simulink model "object"  (R2014a)
settings: Solver=ode45  StartTime=0.0  StopTime=T_sim  FixedStep=0.005  RelTol=1e-3
values from neighbouring files (symbols this model uses):
  Kp = 342.102792836    [all_data.mat]    (also in set_controller_MO.m = Ti/(2*num(end)*Tsig); set_controller_SO.m = T0/(2*K*Tsigma))
  T_sim = 10    [MO_test.m]    (also in SO_test.m; all_data.mat)
  Ti = 0.00201814300939    [all_data.mat]    (also in set_controller_MO.m = T2; set_controller_SO.m = 4*Tsigma)
libraries: cstblocks x1, simulink x1
settings Model: Creator=Gracex  LastModifiedBy=Gracex
settings DebuggingCC: SolverPrmCheckMsg=none

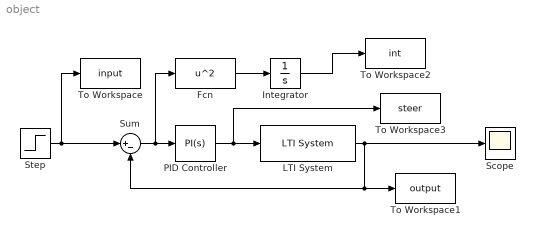
== system object ==
  Fcn : Fcn  Expr=u^2
  Integrator : Integrator
  LTI System : cstblocks/LTI System  sys=G_s  IC=[]
  PID Controller : simulink/Continuous/PID Controller  Controller=PI  TimeDomain=Continuous-time  SampleTime=1  IntegratorMethod=Forward Euler  FilterMethod=Forward Euler  Form=Ideal  P=Kp  I=1/Ti  D=0  N=100  InitialConditionSource=internal  InitialConditionForIntegrator=0  InitialConditionForFilter=0  ExternalReset=none  LimitOutput=off  UpperSaturationLimit=inf  LowerSaturationLimit=-inf  LinearizeAsGain=on  AntiWindupMode=none  Kb=1  TrackingMode=off  Kt=1  PParamMin=[]  PParamMax=[]  IParamMin=[]  IParamMax=[]  DParamMin=[]  DParamMax=[]  NParamMin=[]  NParamMax=[]  KbParamMin=[]  KbParamMax=[]  KtParamMin=[]  KtParamMax=[]  POutMin=[]  POutMax=[]  IOutMin=[]  IOutMax=[]  DOutMin=[]  DOutMax=[]  NOutMin=[]  NOutMax=[]  KbOutMin=[]  KbOutMax=[]  KtOutMin=[]  KtOutMax=[]  IntegratorOutMin=[]  IntegratorOutMax=[]  FilterOutMin=[]  FilterOutMax=[]  SumOutMin=[]  SumOutMax=[]  SumI1OutMin=[]  SumI1OutMax=[]  SumI2OutMin=[]  SumI2OutMax=[]  SumI3OutMin=[]  SumI3OutMax=[]  SumDOutMin=[]  SumDOutMax=[]  SaturationOutMin=[]  SaturationOutMax=[]  IntegratorContinuousStateAttributes=''  IntegratorStateMustResolveToSignalObject=off  IntegratorRTWStateStorageClass=Auto  FilterContinuousStateAttributes=''  FilterStateMustResolveToSignalObject=off  FilterRTWStateStorageClass=Auto
  Scope : Scope
  Step : Step  Time=T_sim/20  SampleTime=0
  Sum : Sum  Inputs=|+-
  To Workspace : ToWorkspace  VariableName=input  SaveFormat=Structure With Time  SampleTime=-1
      settings: Save2DSignal=2-D array (concatenate along first dimension)
  To Workspace1 : ToWorkspace  VariableName=output  SaveFormat=Structure With Time  SampleTime=-1
      settings: Save2DSignal=2-D array (concatenate along first dimension)
  To Workspace2 : ToWorkspace  VariableName=int  SampleTime=-1
      settings: Save2DSignal=2-D array (concatenate along first dimension)
  To Workspace3 : ToWorkspace  VariableName=steer  SaveFormat=Structure With Time  SampleTime=-1
      settings: Save2DSignal=2-D array (concatenate along first dimension)
  wires:
  Step/1 -> Sum/1, To Workspace/1
  LTI System/1 -> Sum/2, To Workspace1/1, Scope/1
  PID Controller/1 -> To Workspace3/1, LTI System/1
  Sum/1 -> Fcn/1, PID Controller/1
  Fcn/1 -> Integrator/1
  Integrator/1 -> To Workspace2/1
